simulink model "VehicleDynamics"  (R2018a)
settings: Solver=VariableStepAuto  StartTime=0.0  StopTime=10.0  RelTol=1e-3
settings Model: Creator=ATRC237_GUO  LastModifiedBy=ATRC237_GUO

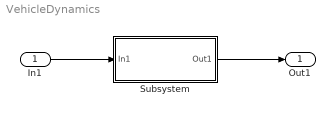
== system VehicleDynamics ==
  In1 : Inport
  Subsystem : Subsystem
  Out1 : Outport
  wires:
  Subsystem/1(Out1) -> Out1/1
  In1/1 -> Subsystem/1(In1)

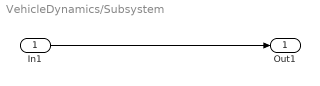
== system VehicleDynamics/Subsystem ==
  In1 : Inport
  Out1 : Outport
  wires:
  In1/1 -> Out1/1
